simulink model "sf_cdplayer"  (R2017b)
settings: Solver=FixedStepDiscrete  StartTime=0.0  StopTime=inf  FixedStep=1  RelTol=1e-3  EnableMultiTasking=on
PreLoadFcn:
  | defaultRadioRequestMode = RadioRequestMode.OFF;
  | defaultCdRequestMode = CdRequestMode.EMPTY;
StartFcn:
  | clear sfcdplayerhelper;
  | sfcdplayergui;
StopFcn:
  | delete(sfcdplayergui);
model workspace (MATLAB code in the model file):
  | Ts = 0.01;  % setup system sample rate
settings Model: Creator=The MathWorks, Inc.  LastModifiedBy=The MathWorks, Inc.
settings DataIOCC: LimitDataPoints=on  SaveFormat=Array  SaveOutput=off  SaveTime=off
settings OptimizationCC: DefaultParameterBehavior=Inlined  ExpressionDepthLimit=2147483647  StateBitsets=on  DataBitsets=on  ZeroExternalMemoryAtStartup=off  ZeroInternalMemoryAtStartup=off  InitFltsAndDblsToZero=on  EfficientFloat2IntCast=on  EfficientMapNaN2IntZero=off  LifeSpan=1
settings DebuggingCC: UnderspecifiedInitializationDetection=Classic  MergeDetectMultiDrivingBlocksExec=none  FcnCallInpInsideContextMsg=warning  AllowSymbolicDim=off  StateNameClashWarn=warning  StrictBusMsg=Warning  SFUnexpectedBacktrackingDiag=warning  SFNoUnconditionalDefaultTransitionDiag=warning  SFExecutionAtInitializationDiag=none
settings HardwareCC: ProdBitPerPointer=32  ProdBitPerSizeT=32  ProdBitPerPtrDiffT=32  ProdLargestAtomicFloat=None  ProdWordSize=32  ProdHWDeviceType=NEC->V850
settings ModelReferenceCC: ModelReferenceNumInstancesAllowed=Single  PropagateSignalLabelsOutOfModel=off
settings SFSimCC: SimParseCustomCode=off
settings RTWCC: SystemTargetFile=ert.tlc  GenCodeOnly=on  TemplateMakefile=ert_default_tmf  Description=Real-Time Workshop Embedded Coder (no auto configuration)  GenerateReport=on  IncludeHyperlinkInReport=on  LaunchReport=on  GenerateTraceInfo=on  GenerateTraceReport=on  GenerateTraceReportSl=on  GenerateTraceReportSf=on  GenerateTraceReportEml=on
settings CodeAppCC: IgnoreCustomStorageClasses=off  CustomSymbolStrType=$N$R$M  CustomSymbolStrModelFcn=$N  StateflowObjectComments=on  InternalIdentifier=Classic
settings ERTTargetCC: MultiwordLength=2048  GenerateSampleERTMain=on  IncludeMdlTerminateFcn=off  SupportAbsoluteTime=off  SupportNonFinite=off  SupportComplex=off  PurelyIntegerCode=on  ERTCustomFileTemplate=example_file_process.tlc  ConvertIfToSwitch=off  SuppressUnreachableDefaultCases=off  EnableUserReplacementTypes=on
settings ConfigComp: CovMetricSettings=dw  CovHtmlReporting=on  CovSaveCumulativeToWorkspaceVar=on  CovSaveSingleToWorkspaceVar=on  CovExternalEMLEnable=off  CovSFcnEnable=off  DVMaxProcessTime=600  DVDisplayUnsatisfiableObjectives=on  DVParameters=on  DVModelCoverageObjectives=MCDC  DVMaxTestCaseSteps=500  DVTestSuiteOptimization=CombinedObjectives  DVDetectActiveLogic=on  DVDetectFloatOverflow=off  DVSaveHarnessModel=on  DVModelReferenceHarness=on  DVSaveReport=on

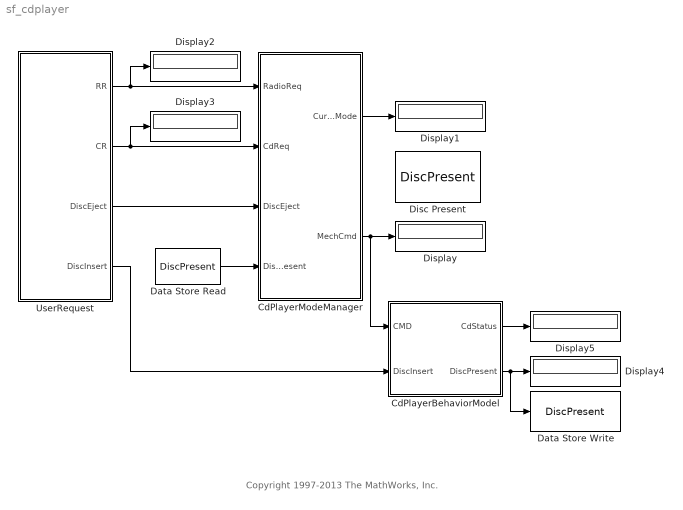
== system sf_cdplayer ==
  note: Copyright 1997-2013 The MathWorks, Inc.
  CdPlayerBehaviorModel : Stateflow chart  TreatAsAtomicUnit=on
  CdPlayerModeManager : Stateflow chart  TreatAsAtomicUnit=on
  Data Store Read : DataStoreRead  DataStoreName=DiscPresent  SampleTime=0
  Data Store Write : DataStoreWrite  DataStoreName=DiscPresent
  Disc Present : DataStoreMemory  DataStoreName=DiscPresent  ShowAdditionalParam=off
  Display{,1..5} (6 alike) : Display
  UserRequest : Stateflow chart  TreatAsAtomicUnit=on
  wires:
  UserRequest/2(CR) -> CdPlayerModeManager/2(CdReq), Display3/1
  Data Store Read/1 -> CdPlayerModeManager/4(DiscPresent)
  CdPlayerModeManager/2(MechCmd) -> Display/1, CdPlayerBehaviorModel/1(CMD)
  CdPlayerModeManager/1(CurrentRadioMode) -> Display1/1
  UserRequest/1(RR) -> CdPlayerModeManager/1(RadioReq), Display2/1
  CdPlayerBehaviorModel/1(CdStatus) -> Display5/1
  CdPlayerBehaviorModel/2(" DiscPresent") -> Data Store Write/1, Display4/1
  UserRequest/4(DiscInsert) -> CdPlayerBehaviorModel/2(DiscInsert)
  UserRequest/3(DiscEject) -> CdPlayerModeManager/3(DiscEject)

== stateflow chart sf_cdplayer/CdPlayerModeManager ==
  state ModeManager
    (history)
    state Standby
      entry: CurrentRadioMode = OFF;
      MechCmd = STOP;
    state ON
      (history)
      state CDMode
        en:
        CurrentRadioMode = CD;
        MechCmd = STOP;
        ex: MechCmd = STOP;
        state Play
          state Normal
            entry: MechCmd = PLAY;
          state Rew
            entry: MechCmd = REW;
          state FastForward
            entry: MechCmd = FF;
          (default) -> Normal
          Play -> Normal [order 3] : [CdReq == PLAY && !in(Normal)]
          Play -> Rew [order 2] : [CdReq == REW && !in(Rew)]
          Play -> FastForward [order 1] : [CdReq == FF && !in(FastForward)]
        state Stop
          entry: MechCmd = STOP;
        (default) -> Play [order 1] : [DiscPresent]
        (default) -> Stop [order 2]
        Play -> Stop [order 1] : [CdReq==STOP]
        Stop -> Play : [DiscPresent && CdReq==PLAY]
      state AMMode
        entry:
        CurrentRadioMode = AM;
        MechCmd = STOP;
      state FMMode
        entry:
        CurrentRadioMode = FM;
        MechCmd = STOP;
      (default) -> (junction 152)
      (junction 152) -> (junction 125)
      (junction 125) -> CDMode [order 1] : [RadioReq==CD]
      ON -> (junction 125) [order 1] : [hasChanged(RadioReq)]
      (junction 125) -> (junction 127) [order 2]
      (junction 127) -> AMMode [order 1] : [RadioReq==AM]
      (junction 127) -> (junction 128) [order 2]
      (junction 128) -> FMMode : /*RadioReq==FM*/
    (default) -> Standby
    Standby -> (junction 152) : [RadioReq != OFF]
    ON -> Standby [order 1] : [RadioReq == OFF]
  state Eject
    entry:
    MechCmd = EJECT;
  (default) -> ModeManager
  ModeManager -> Eject : [DiscEject]
  Eject -> ModeManager
  data: RadioReq input Enum: RadioRequestMode =0xFF; CdReq input Enum: CdRequestMode; DiscEject input; CurrentRadioMode output Enum: RadioRequestMode; DiscPresent input boolean; MechCmd output Enum: CdRequestMode

== stateflow chart sf_cdplayer/UserRequest ==
  (default) -> (junction 13) : {
      | RR = RadioRequestMode(ml.sfcdplayerhelper('get_radio_request'));
      | CR = CdRequestMode(ml.sfcdplayerhelper('get_cd_request'));
      | DiscInsert = ml.sfcdplayerhelper('get_insert_disc');
      | DiscEject = ml.sfcdplayerhelper('get_eject_disc');
      | }
  (junction 13) -> (junction 16)
  data: RR output Enum: RadioRequestMode; CR output Enum: CdRequestMode; DiscEject output boolean; DiscInsert output boolean

== stateflow chart sf_cdplayer/CdPlayerBehaviorModel ==
  state Empty
    CdStatus = EMPTY;
  state Inserting
    CdStatus = DISCINSERT;
  state Ejecting
    CdStatus = EJECT;
  state DiscPresent
    state STOP
      CdStatus = STOP;
    state PLAY
      CdStatus = PLAY;
    state REW
      CdStatus = REW;
    state FF
      CdStatus = FF;
    (default) -> STOP
    DiscPresent -> STOP [order 1] : [CMD == STOP]
    DiscPresent -> PLAY [order 2] : [CMD == PLAY]
    DiscPresent -> REW [order 3] : [CMD == REW]
    DiscPresent -> FF [order 4] : [CMD == FF]
  (default) -> Empty
  Ejecting -> Empty : [after(1/Ts, tick)]
  Empty -> Inserting : [DiscInsert]
  Inserting -> DiscPresent : [after(1/Ts, tick)]
  DiscPresent -> Ejecting [order 1] : [CMD == EJECT]
  data: CMD input; CdStatus output Enum: CdRequestMode; DiscInsert input boolean; Ts parameter; DiscPresent output boolean
